simulink model "bpsk_rx_phase_sync"  (R2019a)
settings: Solver=VariableStepAuto  StartTime=0.0  StopTime=4000/3.2e6  RelTol=1e-3
InitFcn:
  | setup_bpsk_receiver
undefined symbols (not defined in the file): AXI4, designMultirateFIR, Lite, tx_data, xlfda_numerator
libraries: xbsIndex_r4 x172, dspmlti4 x11, hdlsllib x11, dspswit3 x4, dspsigops x2, commrandsrc3 x1, simulink x1
(part 2 of 3)

== system bpsk_rx_phase_sync/Time Synchronisation/NCC ==
  note: For the Numerically Controlled Clock (NCC), we need to consider
      | the symbol oversample factor and the fractional wordlength
      | of the accumulator.
      |
      | The number of samples per symbol determine the maximum value
      | of the accumulator {ceil(log2(n))+1}.
      |
      | The fractional bits determine the quantisation step (precision),
      | of our accumulator.
      |
      | We add 1 to the error signal at all times, as this is necessary to
      | ensure the accumulator always adds 1. If the error is equal to
      | zero, then the accumulator will increase normally. If there is an
      | error in phase not equal to zero, the accumulator will change to
      | compensate for the phase difference.
  Error : Inport
  AddSub : xbsIndex_r4/AddSub  mode=Addition  use_carryin=off  use_carryout=off  en=off  latency=0  precision=User Defined  arith_type=Unsigned  n_bits=n+44  bin_pt=44  quantization=Truncate  overflow=Wrap  use_behavioral_HDL=off  hw_selection=Fabric  pipelined=off  dbl_ovrd=off  block_type=addsub
  AddSub1 : xbsIndex_r4/AddSub  mode=Addition  use_carryin=off  use_carryout=off  en=off  latency=0  precision=Full  arith_type="Signed  (2's comp)"  n_bits=45  bin_pt=44  quantization=Truncate  overflow=Flag as error  use_behavioral_HDL=off  hw_selection=Fabric  pipelined=off  dbl_ovrd=off  block_type=addsub
  Constant : xbsIndex_r4/Constant  const=1  gui_display_data_type=Fixed-point  arith_type=Unsigned  n_bits=1  bin_pt=0  preci_type=Single  exp_width=8  frac_width=24  explicit_period=off  period=1  equ=P=C  opselect=C  inp2=PCIN>>17  opr=+  inp1=P  carry=CIN  dbl_ovrd=off  block_type=constant
  Register : xbsIndex_r4/Register  init=0  rst=off  en=off  dbl_ovrd=off  block_type=register
  Relational : xbsIndex_r4/Relational  mode=a<b  op_type=Bool  en=off  latency=0  dbl_ovrd=off  block_type=relational
  Strobe : Outport
  wires:
  Register/1 -> AddSub/1, Relational/2
  Relational/1 -> Strobe/1
  AddSub/1 -> Register/1, Relational/1
  AddSub1/1 -> AddSub/2
  Constant/1 -> AddSub1/1
  Error/1 -> AddSub1/2

== system bpsk_rx_phase_sync/Time Synchronisation/Timing Error Detector ==
  Real In : Inport
  Imag In : Inport  Port=2
  AddSub : xbsIndex_r4/AddSub  mode=Subtraction  use_carryin=off  use_carryout=off  en=off  latency=0  precision=Full  arith_type=Unsigned  n_bits=16  bin_pt=14  quantization=Truncate  overflow=Wrap  use_behavioral_HDL=off  hw_selection=Fabric  pipelined=off  dbl_ovrd=off  block_type=addsub
  AddSub1 : xbsIndex_r4/AddSub  mode=Subtraction  use_carryin=off  use_carryout=off  en=off  latency=0  precision=Full  arith_type=Unsigned  n_bits=16  bin_pt=14  quantization=Truncate  overflow=Wrap  use_behavioral_HDL=off  hw_selection=Fabric  pipelined=off  dbl_ovrd=off  block_type=addsub
  AddSub2 : xbsIndex_r4/AddSub  mode=Addition  use_carryin=off  use_carryout=off  en=off  latency=0  precision=Full  arith_type="Signed  (2's comp)"  n_bits=33  bin_pt=25  quantization="Round  (unbiased: +/- Inf)"  overflow=Saturate  use_behavioral_HDL=off  hw_selection=Fabric  pipelined=off  dbl_ovrd=off  block_type=addsub
  Delay : xbsIndex_r4/Delay  rst=off  infoeditControl=Selection of Reset will increase slice count due to use of real FFs and instead of SRLs  en=off  latency=32  reg_retiming=off  dbl_ovrd=off  block_type=delay
  Delay1 : xbsIndex_r4/Delay  rst=off  infoeditControl=Selection of Reset will increase slice count due to use of real FFs and instead of SRLs  en=off  latency=32  reg_retiming=off  dbl_ovrd=off  block_type=delay
  Mult1 : xbsIndex_r4/Mult  precision=Full  arith_type=Unsigned  n_bits=31  bin_pt=28  quantization=Truncate  overflow=Saturate  en=off  latency=0  use_behavioral_HDL=off  opt=Speed  use_embedded=on  optimum_pipeline=off  pipeline=on  dbl_ovrd=off  use_rpm=on  placement_style=Triangular  block_type=mult
  Mult2 : xbsIndex_r4/Mult  precision=Full  arith_type=Unsigned  n_bits=31  bin_pt=28  quantization=Truncate  overflow=Saturate  en=off  latency=0  use_behavioral_HDL=off  opt=Speed  use_embedded=on  optimum_pipeline=off  pipeline=on  dbl_ovrd=off  use_rpm=on  placement_style=Triangular  block_type=mult
  Error : Outport
  wires:
  Real In/1 -> Mult1/1, Mult1/2
  Imag In/1 -> Mult2/1, Mult2/2
  AddSub/1 -> AddSub2/1
  AddSub2/1 -> Error/1
  Delay1/1 -> AddSub1/2
  Mult2/1 -> Delay1/1, AddSub1/1
  AddSub1/1 -> AddSub2/2
  Mult1/1 -> AddSub/1, Delay/1
  Delay/1 -> AddSub/2

== system bpsk_rx_phase_sync/BPSK System/BPSK RX Generation/RRC Receive Filter ==
  Data In : Inport
  Data Type Conversion2 : DataTypeConversion  OutDataTypeStr=fixdt(1,16,14)
  FDATool : xbsIndex_r4/FDATool  block_type=fdatool
      settings: infoedit=FDATool
  FIR Decimation : dspmlti4/FIR Decimation  FilterSource=Dialog parameters  h=xlfda_numerator('FDATool')/(max(xlfda_numerator('FDATool'))*4)  D=4  filtStruct=Direct form  FilterObject=FDECIM  framing=Allow multirate processing  inputOffset=0  outputBufInitCond=0  roundingMode=Floor  overflowMode=off  firstCoeffMode=Binary point scaling  firstCoeffWordLength=16  firstCoeffFracLength=14  firstCoeffDataTypeStr=fixdt(1,16,14)  firstCoeffMin=[]  firstCoeffMax=[]  firstCoeffLastDataTypeStr=fixdt(1,16,14)  outputDataTypeStr=Inherit: Same as accumulator  outputMin=[]  outputMax=[]  outputLastDataTypeStr=Inherit: Same as accumulator
  Data Out : Outport
  wires:
  FIR Decimation/1 -> Data Type Conversion2/1
  Data In/1 -> FIR Decimation/1
  Data Type Conversion2/1 -> Data Out/1

== system bpsk_rx_phase_sync/BPSK System/BPSK TX Generation/DBPSK Modulator ==
  Input : Inport
  Cast To Boolean : DataTypeConversion  OutDataTypeStr=boolean
  Constant : Constant  Value=fi(1, 1, 16, 14)  OutDataTypeStr=fixdt(1,16,14)  SampleTime=-1
  Constant1 : Constant  Value=fi(-1, 1, 16, 14)  OutDataTypeStr=fixdt(1,16,14)  SampleTime=-1
  Constant2 : Constant  Value=0  OutDataTypeStr=Inherit: Inherit via back propagation  SampleTime=-1
  Delay : Delay  DelayLength=1
  Multiport Switch : MultiPortSwitch  DataPortOrder=Zero-based contiguous  Inputs=2  zeroidx=on
  Real-Imag to Complex : RealImagToComplex
  XOR : Logic  Operator=XOR  IconShape=distinctive  AllPortsSameDT=off  OutDataTypeStr=boolean
  Output : Outport
  wires:
  Constant2/1 -> Real-Imag to Complex/2
  Real-Imag to Complex/1 -> Output/1
  Multiport Switch/1 -> Real-Imag to Complex/1
  Constant1/1 -> Multiport Switch/3
  Constant/1 -> Multiport Switch/2
  Input/1 -> Cast To Boolean/1
  Delay/1 -> XOR/1
  XOR/1 -> Multiport Switch/1, Delay/1
  Cast To Boolean/1 -> XOR/2

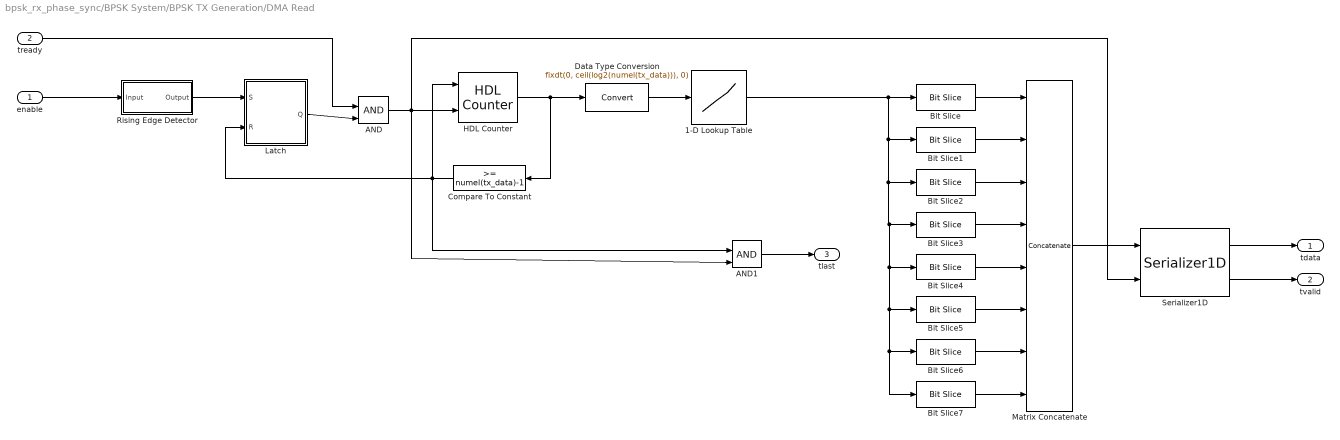
== system bpsk_rx_phase_sync/BPSK System/BPSK TX Generation/DMA Read ==
  enable : Inport
  tready : Inport  Port=2
  1-D Lookup Table : Lookup_n-D  NumberOfTableDimensions=1  BreakpointsForDimension1=[0:1:numel(tx_data)-1]  Table=tx_data  TableDataTypeStr=Inherit: Inherit from 'Table data'  ExtrapMethod=Clip  InternalRulePriority=Speed  OutDataTypeStr=Inherit: Inherit from 'Table data'  RndMeth=Simplest  InputSameDT=on
  AND : Logic  IconShape=distinctive  AllPortsSameDT=off  OutDataTypeStr=boolean
  AND1 : Logic  IconShape=distinctive  AllPortsSameDT=off  OutDataTypeStr=boolean
  Bit Slice : hdlsllib/Logic and Bit Operations/Bit Slice  lidx=0  ridx=0
      settings: SourceProductName=Simulink  SourceProductBaseCode=SL
  Bit Slice1 : hdlsllib/Logic and Bit Operations/Bit Slice  lidx=1  ridx=1
      settings: SourceProductName=Simulink  SourceProductBaseCode=SL
  Bit Slice2 : hdlsllib/Logic and Bit Operations/Bit Slice  lidx=2  ridx=2
      settings: SourceProductName=Simulink  SourceProductBaseCode=SL
  Bit Slice3 : hdlsllib/Logic and Bit Operations/Bit Slice  lidx=3  ridx=3
      settings: SourceProductName=Simulink  SourceProductBaseCode=SL
  Bit Slice4 : hdlsllib/Logic and Bit Operations/Bit Slice  lidx=4  ridx=4
      settings: SourceProductName=Simulink  SourceProductBaseCode=SL
  Bit Slice5 : hdlsllib/Logic and Bit Operations/Bit Slice  lidx=5  ridx=5
      settings: SourceProductName=Simulink  SourceProductBaseCode=SL
  Bit Slice6 : hdlsllib/Logic and Bit Operations/Bit Slice  lidx=6  ridx=6
      settings: SourceProductName=Simulink  SourceProductBaseCode=SL
  Bit Slice7 : hdlsllib/Logic and Bit Operations/Bit Slice  lidx=7  ridx=7
      settings: SourceProductName=Simulink  SourceProductBaseCode=SL
  Compare To Constant : simulink/Logic and Bit Operations/Compare To Constant  relop=>=  const=numel(tx_data)-1  OutDataTypeStr=boolean
  Data Type Conversion : DataTypeConversion  OutDataTypeStr=fixdt(0, ceil(log2(numel(tx_data))), 0)
  HDL Counter : hdlsllib/Sources/HDL Counter  CountType=Free running  CountInit=0  CountStep=1  CountMax=25  CountFromType=Initial value  CountFrom=0  CountResetPort=on  CountLoadPort=off  CountEnbPort=on  CountDirPort=off  CountDataType=Unsigned  CountWordLen=32  CountFracLen=0  CountSampTime=1
      settings: SourceProductName=Simulink
  Latch : Subsystem
  Matrix Concatenate : Concatenate  NumInputs=8  Mode=Multidimensional array  ConcatenateDimension=2
  Rising Edge Detector : Subsystem
  Serializer1D : hdlsllib/HDL Operations/Serializer1D  Ratio=8  IdleCycles=0  validIn=on  startOut=off  validOut=on  inputDataDimensions=-1  inputSampleTime=-1  inputSignalType=auto
      settings: SourceProductName=Simulink  SourceProductBaseCode=SL
  tdata : Outport
  tvalid : Outport  Port=2
  tlast : Outport  Port=3
  wires:
  Serializer1D/2 -> tvalid/1
  Bit Slice5/1 -> Matrix Concatenate/6
  Bit Slice6/1 -> Matrix Concatenate/7
  Bit Slice7/1 -> Matrix Concatenate/8
  Bit Slice4/1 -> Matrix Concatenate/5
  Serializer1D/1 -> tdata/1
  1-D Lookup Table/1 -> Bit Slice/1, Bit Slice1/1, Bit Slice2/1, Bit Slice3/1, Bit Slice4/1, Bit Slice5/1, Bit Slice6/1, Bit Slice7/1
  Bit Slice2/1 -> Matrix Concatenate/3
  Bit Slice1/1 -> Matrix Concatenate/2
  Bit Slice3/1 -> Matrix Concatenate/4
  Bit Slice/1 -> Matrix Concatenate/1
  Matrix Concatenate/1 -> Serializer1D/1
  Compare To Constant/1 -> AND1/1, HDL Counter/1, Latch/2(R)
  enable/1 -> Rising Edge Detector/1(Input)
  HDL Counter/1 -> Compare To Constant/1, Data Type Conversion/1
  Data Type Conversion/1 -> 1-D Lookup Table/1
  Rising Edge Detector/1(Output) -> Latch/1(S)
  AND/1 -> AND1/2, Serializer1D/2, HDL Counter/2
  Latch/1(Q) -> AND/2
  tready/1 -> AND/1
  AND1/1 -> tlast/1

== system bpsk_rx_phase_sync/BPSK System/RF-ADC/Decimation Filter ==
  Data In : Inport
  FIR 0 : dspmlti4/FIR Decimation  FilterSource=Filter object  h=designMultirateFIR(1,2)  D=2  filtStruct=Direct form  FilterObject=fir0  InputProcessing=Columns as channels (frame based)  framing=Allow multirate processing  inputOffset=0  outputBufInitCond=0  roundingMode=Floor  overflowMode=off  firstCoeffDataTypeStr=Inherit: Same word length as input  firstCoeffMin=[]  firstCoeffMax=[]  firstCoeffLastDataTypeStr=Inherit: Same word length as input  outputDataTypeStr=Inherit: Same as accumulator  outputMin=[]  outputMax=[]  outputLastDataTypeStr=Inherit: Same as accumulator
  FIR 1 : dspmlti4/FIR Decimation  FilterSource=Filter object  h=designMultirateFIR(1,2)  D=2  filtStruct=Direct form  FilterObject=fir1  InputProcessing=Columns as channels (frame based)  framing=Allow multirate processing  inputOffset=0  outputBufInitCond=0  roundingMode=Floor  overflowMode=off  firstCoeffDataTypeStr=Inherit: Same word length as input  firstCoeffMin=[]  firstCoeffMax=[]  firstCoeffLastDataTypeStr=Inherit: Same word length as input  outputDataTypeStr=Inherit: Same as accumulator  outputMin=[]  outputMax=[]  outputLastDataTypeStr=Inherit: Same as accumulator
  FIR 2 : dspmlti4/FIR Decimation  FilterSource=Filter object  h=designMultirateFIR(1,2)  D=2  filtStruct=Direct form  FilterObject=fir2  InputProcessing=Columns as channels (frame based)  framing=Allow multirate processing  inputOffset=0  outputBufInitCond=0  roundingMode=Floor  overflowMode=off  firstCoeffDataTypeStr=Inherit: Same word length as input  firstCoeffMin=[]  firstCoeffMax=[]  firstCoeffLastDataTypeStr=Inherit: Same word length as input  outputDataTypeStr=Inherit: Same as accumulator  outputMin=[]  outputMax=[]  outputLastDataTypeStr=Inherit: Same as accumulator
  Data Out : Outport
  wires:
  FIR 2/1 -> FIR 1/1
  Data In/1 -> FIR 2/1
  FIR 0/1 -> Data Out/1
  FIR 1/1 -> FIR 0/1

== system bpsk_rx_phase_sync/BPSK System/RF-ADC/NCO and Mixer ==
  Data In : Inport
  Constant1 : Constant  Value=m  OutDataTypeStr=fixdt(0,2,0)  SampleTime=-1
  Data Type Conversion : DataTypeConversion  OutDataTypeStr=fixdt(1,16,14)
  Multiport Switch1 : MultiPortSwitch  DataPortOrder=Zero-based contiguous  zeroidx=on
  RF-ADC Coarse Mixer : Subsystem
  RF-ADC Fine Mixer : Subsystem
  Real-Imag to Complex : RealImagToComplex
  Data Out : Outport
  wires:
  Data Type Conversion/1 -> Multiport Switch1/2
  Constant1/1 -> Multiport Switch1/1
  Data In/1 -> Real-Imag to Complex/2, RF-ADC Fine Mixer/1(Data In), RF-ADC Coarse Mixer/1(Data In), Real-Imag to Complex/1
  RF-ADC Coarse Mixer/1(Data Out) -> Multiport Switch1/3
  Real-Imag to Complex/1 -> Data Type Conversion/1
  RF-ADC Fine Mixer/1(Data Out) -> Multiport Switch1/4
  Multiport Switch1/1 -> Data Out/1

== system bpsk_rx_phase_sync/BPSK System/RF-ADC/RF-ADC ==
  Data In : Inport
  Buffer : Buffer  N=ssr  OutputFrames=off
  Data Type Conversion : DataTypeConversion  OutDataTypeStr=fixdt(1,12,10)
  Rate Transition : RateTransition  OutPortSampleTime=1/fs
  Data Out : Outport
  wires:
  Buffer/1 -> Data Out/1
  Data Type Conversion/1 -> Buffer/1
  Data In/1 -> Rate Transition/1
  Rate Transition/1 -> Data Type Conversion/1

== system bpsk_rx_phase_sync/BPSK System/RF-DAC/Coarse Delay ==
  Data In : Inport
  Data Out : Outport
  wires:
  Data In/1 -> Data Out/1

== system bpsk_rx_phase_sync/BPSK System/RF-DAC/Interpolation Filter ==
  Data In : Inport
  FIR 0 : dspmlti4/FIR Interpolation  FilterSource=Filter object  h=designMultirateFIR(3,1)  L=2  FilterObject=fir0  InputProcessing=Columns as channels (frame based)  framing=Allow multirate processing  outputBufInitCond=0  roundingMode=Floor  overflowMode=off  firstCoeffDataTypeStr=Inherit: Same word length as input  firstCoeffMin=[]  firstCoeffMax=[]  firstCoeffLastDataTypeStr=Inherit: Same word length as input  outputDataTypeStr=Inherit: Same as accumulator  outputMin=[]  outputMax=[]  outputLastDataTypeStr=Inherit: Same as accumulator
      settings: SourceProductName=DSP System Toolbox
  FIR 1 : dspmlti4/FIR Interpolation  FilterSource=Filter object  h=designMultirateFIR(3,1)  L=2  FilterObject=fir1  InputProcessing=Columns as channels (frame based)  framing=Allow multirate processing  outputBufInitCond=0  roundingMode=Floor  overflowMode=off  firstCoeffDataTypeStr=Inherit: Same word length as input  firstCoeffMin=[]  firstCoeffMax=[]  firstCoeffLastDataTypeStr=Inherit: Same word length as input  outputDataTypeStr=Inherit: Same as accumulator  outputMin=[]  outputMax=[]  outputLastDataTypeStr=Inherit: Same as accumulator
      settings: SourceProductName=DSP System Toolbox
  FIR 2 : dspmlti4/FIR Interpolation  FilterSource=Filter object  h=designMultirateFIR(3,1)  L=2  FilterObject=fir2  InputProcessing=Columns as channels (frame based)  framing=Allow multirate processing  outputBufInitCond=0  roundingMode=Floor  overflowMode=off  firstCoeffDataTypeStr=Inherit: Same word length as input  firstCoeffMin=[]  firstCoeffMax=[]  firstCoeffLastDataTypeStr=Inherit: Same word length as input  outputDataTypeStr=Inherit: Same as accumulator  outputMin=[]  outputMax=[]  outputLastDataTypeStr=Inherit: Same as accumulator
      settings: SourceProductName=DSP System Toolbox
  Data Out : Outport
  wires:
  FIR 1/1 -> FIR 0/1
  FIR 0/1 -> Data Out/1
  Data In/1 -> FIR 2/1
  FIR 2/1 -> FIR 1/1

== system bpsk_rx_phase_sync/BPSK System/RF-DAC/NCO and Mixer ==
  Data In : Inport
  Complex to Real-Imag : ComplexToRealImag
  Constant1 : Constant  Value=m  OutDataTypeStr=fixdt(0,2,0)  SampleTime=-1
  Multiport Switch1 : MultiPortSwitch  DataPortOrder=Zero-based contiguous  zeroidx=on
  RF-DAC Coarse Mixer : Subsystem
  RF-DAC Fine Mixer : Subsystem
  Terminator : Terminator
  Data Out : Outport
  wires:
  Complex to Real-Imag/2 -> Terminator/1
  Complex to Real-Imag/1 -> Multiport Switch1/2
  RF-DAC Fine Mixer/1(Data Out) -> Multiport Switch1/4
  Multiport Switch1/1 -> Data Out/1
  Data In/1 -> RF-DAC Fine Mixer/1(Data In), RF-DAC Coarse Mixer/1(Data In), Complex to Real-Imag/1
  Constant1/1 -> Multiport Switch1/1
  RF-DAC Coarse Mixer/1(Data Out) -> Multiport Switch1/3

== system bpsk_rx_phase_sync/BPSK System/RF-DAC/Output Filter ==
  Data In : Inport
  Data Out : Outport
  wires:
  Data In/1 -> Data Out/1

== system bpsk_rx_phase_sync/BPSK System/RF-DAC/QMC Gain & Phase ==
  Data In : Inport
  Data Out : Outport
  wires:
  Data In/1 -> Data Out/1

== system bpsk_rx_phase_sync/BPSK System/RF-DAC/QMC Threshold ==
  Data In : Inport
  Data Out : Outport
  wires:
  Data In/1 -> Data Out/1

== system bpsk_rx_phase_sync/BPSK System/RF-DAC/RF-DAC ==
  Data In : Inport
  Cast To Double : DataTypeConversion  OutDataTypeStr=double
  Rate Transition : RateTransition  OutPortSampleTime=0
  Unbuffer : Unbuffer
  Data Out : Outport
  wires:
  Rate Transition/1 -> Data Out/1
  Data In/1 -> Unbuffer/1
  Unbuffer/1 -> Cast To Double/1
  Cast To Double/1 -> Rate Transition/1

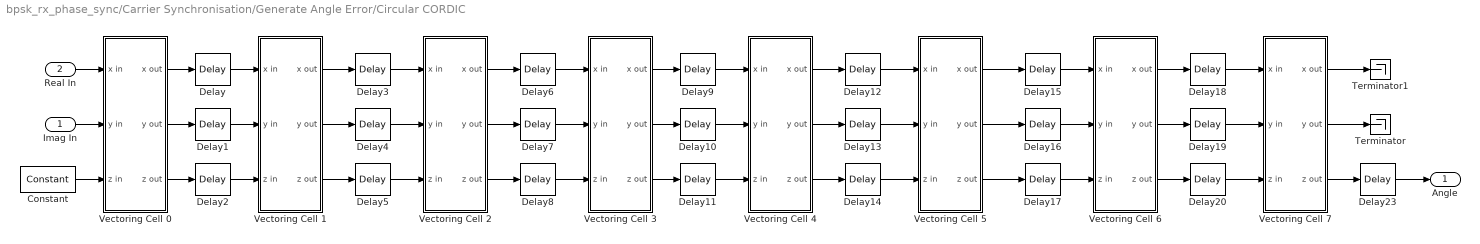
== system bpsk_rx_phase_sync/Carrier Synchronisation/Generate Angle Error/Circular CORDIC ==
  Imag In : Inport
  Real In : Inport  Port=2
  Constant : xbsIndex_r4/Constant  const=0  gui_display_data_type=Fixed-point  arith_type=Signed (2's comp)  n_bits=16  bin_pt=14  preci_type=Single  exp_width=8  frac_width=24  explicit_period=off  period=1  equ=P=C  opselect=C  inp2=PCIN>>17  opr=+  inp1=P  carry=CIN  dbl_ovrd=off  block_type=constant
  Delay{,1..20,23} (22 alike) : xbsIndex_r4/Delay  rst=off  infoeditControl=Selection of Reset will increase slice count due to use of real FFs and instead of SRLs  en=off  latency=1  reg_retiming=off  dbl_ovrd=off  block_type=delay
  Terminator : Terminator
  Terminator1 : Terminator
  Vectoring Cell 0 : Subsystem  mask(Cordic Vectoring Cell){i=0}
      mask prompts: i "Iteration:"
      mask help: some notes to go here
      mask DialogControl DescGroupVar Prompt: CORDIC Vectoring Cell
      mask DialogControl DescTextVar Prompt: A single cell of a vectoring CORDIC unrolled architecture.
      mask DialogControl ParameterGroupVar Prompt: Main
  Vectoring Cell 1 : Subsystem  mask(Cordic Vectoring Cell){i=1}
      mask prompts: i "Iteration:"
      mask help: some notes to go here
      mask DialogControl DescGroupVar Prompt: CORDIC Vectoring Cell
      mask DialogControl DescTextVar Prompt: A single cell of a vectoring CORDIC unrolled architecture.
      mask DialogControl ParameterGroupVar Prompt: Main
  Vectoring Cell 2 : Subsystem  mask(Cordic Vectoring Cell){i=2}
      mask prompts: i "Iteration:"
      mask help: some notes to go here
      mask DialogControl DescGroupVar Prompt: CORDIC Vectoring Cell
      mask DialogControl DescTextVar Prompt: A single cell of a vectoring CORDIC unrolled architecture.
      mask DialogControl ParameterGroupVar Prompt: Main
  Vectoring Cell 3 : Subsystem  mask(Cordic Vectoring Cell){i=3}
      mask prompts: i "Iteration:"
      mask help: some notes to go here
      mask DialogControl DescGroupVar Prompt: CORDIC Vectoring Cell
      mask DialogControl DescTextVar Prompt: A single cell of a vectoring CORDIC unrolled architecture.
      mask DialogControl ParameterGroupVar Prompt: Main
  Vectoring Cell 4 : Subsystem  mask(Cordic Vectoring Cell){i=4}
      mask prompts: i "Iteration:"
      mask help: some notes to go here
      mask DialogControl DescGroupVar Prompt: CORDIC Vectoring Cell
      mask DialogControl DescTextVar Prompt: A single cell of a vectoring CORDIC unrolled architecture.
      mask DialogControl ParameterGroupVar Prompt: Main
  Vectoring Cell 5 : Subsystem  mask(Cordic Vectoring Cell){i=5}
      mask prompts: i "Iteration:"
      mask help: some notes to go here
      mask DialogControl DescGroupVar Prompt: CORDIC Vectoring Cell
      mask DialogControl DescTextVar Prompt: A single cell of a vectoring CORDIC unrolled architecture.
      mask DialogControl ParameterGroupVar Prompt: Main
  Vectoring Cell 6 : Subsystem  mask(Cordic Vectoring Cell){i=6}
      mask prompts: i "Iteration:"
      mask help: some notes to go here
      mask DialogControl DescGroupVar Prompt: CORDIC Vectoring Cell
      mask DialogControl DescTextVar Prompt: A single cell of a vectoring CORDIC unrolled architecture.
      mask DialogControl ParameterGroupVar Prompt: Main
  Vectoring Cell 7 : Subsystem  mask(Cordic Vectoring Cell){i=7}
      mask prompts: i "Iteration:"
      mask help: some notes to go here
      mask DialogControl DescGroupVar Prompt: CORDIC Vectoring Cell
      mask DialogControl DescTextVar Prompt: A single cell of a vectoring CORDIC unrolled architecture.
      mask DialogControl ParameterGroupVar Prompt: Main
  Angle : Outport
  wires:
  Vectoring Cell 6/3(z out) -> Delay20/1
  Delay5/1 -> Vectoring Cell 2/3(z in)
  Vectoring Cell 6/2(y out) -> Delay19/1
  Vectoring Cell 2/1(x out) -> Delay6/1
  Vectoring Cell 1/3(z out) -> Delay5/1
  Delay14/1 -> Vectoring Cell 5/3(z in)
  Delay20/1 -> Vectoring Cell 7/3(z in)
  Delay15/1 -> Vectoring Cell 6/1(x in)
  Delay7/1 -> Vectoring Cell 3/2(y in)
  Delay1/1 -> Vectoring Cell 1/2(y in)
  Vectoring Cell 3/1(x out) -> Delay9/1
  Delay13/1 -> Vectoring Cell 5/2(y in)
  Delay9/1 -> Vectoring Cell 4/1(x in)
  Vectoring Cell 1/1(x out) -> Delay3/1
  Delay16/1 -> Vectoring Cell 6/2(y in)
  Delay18/1 -> Vectoring Cell 7/1(x in)
  Vectoring Cell 0/3(z out) -> Delay2/1
  Delay10/1 -> Vectoring Cell 4/2(y in)
  Vectoring Cell 2/2(y out) -> Delay7/1
  Vectoring Cell 3/3(z out) -> Delay11/1
  Delay6/1 -> Vectoring Cell 3/1(x in)
  Delay19/1 -> Vectoring Cell 7/2(y in)
  Delay4/1 -> Vectoring Cell 2/2(y in)
  Delay3/1 -> Vectoring Cell 2/1(x in)
  Vectoring Cell 4/3(z out) -> Delay14/1
  Delay8/1 -> Vectoring Cell 3/3(z in)
  Vectoring Cell 3/2(y out) -> Delay10/1
  Vectoring Cell 1/2(y out) -> Delay4/1
  Vectoring Cell 5/1(x out) -> Delay15/1
  Delay/1 -> Vectoring Cell 1/1(x in)
  Vectoring Cell 5/2(y out) -> Delay16/1
  Vectoring Cell 0/1(x out) -> Delay/1
  Vectoring Cell 2/3(z out) -> Delay8/1
  Vectoring Cell 6/1(x out) -> Delay18/1
  Vectoring Cell 0/2(y out) -> Delay1/1
  Delay12/1 -> Vectoring Cell 5/1(x in)
  Vectoring Cell 4/2(y out) -> Delay13/1
  Vectoring Cell 4/1(x out) -> Delay12/1
  Delay2/1 -> Vectoring Cell 1/3(z in)
  Vectoring Cell 5/3(z out) -> Delay17/1
  Delay17/1 -> Vectoring Cell 6/3(z in)
  Delay11/1 -> Vectoring Cell 4/3(z in)
  Vectoring Cell 7/3(z out) -> Delay23/1
  Real In/1 -> Vectoring Cell 0/1(x in)
  Imag In/1 -> Vectoring Cell 0/2(y in)
  Constant/1 -> Vectoring Cell 0/3(z in)
  Delay23/1 -> Angle/1
  Vectoring Cell 7/2(y out) -> Terminator/1
  Vectoring Cell 7/1(x out) -> Terminator1/1

== system bpsk_rx_phase_sync/Carrier Synchronisation/Generate NCO/Loop Filter ==
  Signal : Inport
  Strobe : Inport  Port=2
  Reset : Inport  Port=3
  AddSub : xbsIndex_r4/AddSub  mode=Addition  use_carryin=off  use_carryout=off  en=off  latency=0  precision=User Defined  arith_type="Signed  (2's comp)"  n_bits=36  bin_pt=34  quantization=Truncate  overflow=Flag as error  use_behavioral_HDL=off  hw_selection=Fabric  pipelined=off  dbl_ovrd=off  block_type=addsub
  AddSub1 : xbsIndex_r4/AddSub  mode=Addition  use_carryin=off  use_carryout=off  en=off  latency=0  precision=Full  arith_type="Signed  (2's comp)"  n_bits=32  bin_pt=31  quantization=Truncate  overflow=Wrap  use_behavioral_HDL=off  hw_selection=Fabric  pipelined=off  dbl_ovrd=off  block_type=addsub
  K1_Gain : xbsIndex_r4/CMult  const=K1  gui_display_data_type=Fixed-point  const_n_bits=16  const_bin_pt=16  float_type=Single  exp_bits=8  fraction_bits=24  en=off  latency=0  precision=Full  arith_type="Signed  (2's comp)"  n_bits=20  bin_pt=14  quantization=Truncate  overflow=Wrap  use_behavioral_HDL=off  mem_type=Distributed RAM  pipeline=off  dbl_ovrd=off  block_type=cmult
  K2_Gain : xbsIndex_r4/CMult  const=K2  gui_display_data_type=Fixed-point  const_n_bits=16  const_bin_pt=16  float_type=Single  exp_bits=8  fraction_bits=24  en=off  latency=0  precision=Full  arith_type="Signed  (2's comp)"  n_bits=20  bin_pt=14  quantization=Truncate  overflow=Wrap  use_behavioral_HDL=off  mem_type=Distributed RAM  pipeline=off  dbl_ovrd=off  block_type=cmult
  Register : xbsIndex_r4/Register  init=0  rst=on  en=on  dbl_ovrd=off  block_type=register
  Register1 : xbsIndex_r4/Register  init=0  rst=on  en=on  dbl_ovrd=off  block_type=register
  Register3 : xbsIndex_r4/Register  init=0  rst=off  en=off  dbl_ovrd=off  block_type=register
  Register4 : xbsIndex_r4/Register  init=0  rst=off  en=off  dbl_ovrd=off  block_type=register
  Error : Outport
  Valid : Outport  Port=2
  wires:
  Reset/1 -> Register/2, Register1/2
  Signal/1 -> Register1/1
  K2_Gain/1 -> AddSub/1
  AddSub/1 -> AddSub1/2, Register/1
  Register/1 -> AddSub/2
  Register1/1 -> K2_Gain/1, K1_Gain/1
  AddSub1/1 -> Register3/1
  K1_Gain/1 -> AddSub1/1
  Register3/1 -> Error/1
  Register4/1 -> Valid/1
  Strobe/1 -> Register4/1, Register/3, Register1/3

== system bpsk_rx_phase_sync/Carrier Synchronisation/Generate NCO/NCO ==
  Step Size : Inport
  En_in : Inport  Port=2
  AddSub4 : xbsIndex_r4/AddSub  mode=Addition  use_carryin=off  use_carryout=off  en=off  latency=0  precision=User Defined  arith_type="Signed  (2's comp)"  n_bits=n+b  bin_pt=b  quantization=Truncate  overflow=Wrap  use_behavioral_HDL=off  hw_selection=Fabric  pipelined=off  dbl_ovrd=off  block_type=addsub
  CMult1 : xbsIndex_r4/CMult  const=(2^n)/(2*pi)  gui_display_data_type=Fixed-point  const_n_bits=k_n+b  const_bin_pt=b  float_type=Single  exp_bits=8  fraction_bits=24  en=off  latency=0  precision=User Defined  arith_type="Signed  (2's comp)"  n_bits=n+b  bin_pt=b  quantization=Truncate  overflow=Wrap  use_behavioral_HDL=off  mem_type=Distributed RAM  pipeline=off  dbl_ovrd=off  block_type=cmult
  Convert1 : xbsIndex_r4/Convert  gui_display_data_type=Fixed-point  arith_type=Unsigned  n_bits=n  bin_pt=0  float_type=Single  exp_bits=8  fraction_bits=24  quantization=Truncate  overflow=Wrap  en=off  latency=0  pipeline=off  dbl_ovrd=off  block_type=convert
  Cos ROM : xbsIndex_r4/ROM  depth=2^n  initVector=cos(pi*(0:((2^n)-1))/(2^(n-1)))  distributed_mem=Block RAM  rst=off  init_reg=0  en=off  latency=1  gui_display_data_type=Fixed-point  arith_type="Signed  (2's comp)"  n_bits=16  bin_pt=14  preci_type=Single  exp_width=8  frac_width=24  optimize=Area  use_rpm=on  dbl_ovrd=off  block_type=sprom
  Neg Sin ROM : xbsIndex_r4/ROM  depth=2^n  initVector=-sin(pi*(0:((2^n)-1))/(2^(n-1)))  distributed_mem=Block RAM  rst=off  init_reg=0  en=off  latency=1  gui_display_data_type=Fixed-point  arith_type="Signed  (2's comp)"  n_bits=16  bin_pt=14  preci_type=Single  exp_width=8  frac_width=24  optimize=Area  use_rpm=on  dbl_ovrd=off  block_type=sprom
  Register : xbsIndex_r4/Register  init=0  rst=off  en=off  dbl_ovrd=off  block_type=register
  Register1 : xbsIndex_r4/Register  init=0  rst=off  en=on  dbl_ovrd=off  block_type=register
  Cos : Outport
  Neg Sin : Outport  Port=2
  En_out : Outport  Port=3
  wires:
  Convert1/1 -> Neg Sin ROM/1, Cos ROM/1
  AddSub4/1 -> Register1/1, Convert1/1
  Neg Sin ROM/1 -> Neg Sin/1
  Register1/1 -> AddSub4/2
  CMult1/1 -> AddSub4/1
  Step Size/1 -> CMult1/1
  En_in/1 -> Register/1, Register1/2
  Cos ROM/1 -> Cos/1
  Register/1 -> En_out/1

== system bpsk_rx_phase_sync/BPSK System/BPSK TX Generation/DMA Read/Latch ==
  S : Inport
  R : Inport  Port=2
  Multiport Switch : MultiPortSwitch  DataPortOrder=Zero-based contiguous  Inputs=2  zeroidx=on
  Unit Delay Resettable Synchronous : hdlsllib/Discrete/Unit Delay Resettable Synchronous  InitialCondition=0.0  SampleTime=-1
      settings: SourceProductName=Simulink  SourceProductBaseCode=SL
  Q : Outport
  wires:
  Multiport Switch/1 -> Unit Delay Resettable Synchronous/1, Q/1
  S/1 -> Multiport Switch/3, Multiport Switch/1
  Unit Delay Resettable Synchronous/1 -> Multiport Switch/2
  R/1 -> Unit Delay Resettable Synchronous/2

== system bpsk_rx_phase_sync/BPSK System/BPSK TX Generation/DMA Read/Rising Edge Detector ==
  Input : Inport
  AND1 : Logic  IconShape=distinctive  AllPortsSameDT=off  OutDataTypeStr=boolean
  Delay1 : Delay  DelayLength=1
  NOT : Logic  Operator=NOT  IconShape=distinctive  AllPortsSameDT=off  OutDataTypeStr=boolean
  Output : Outport
  wires:
  NOT/1 -> AND1/1
  Input/1 -> AND1/2, Delay1/1
  Delay1/1 -> NOT/1
  AND1/1 -> Output/1

== system bpsk_rx_phase_sync/BPSK System/RF-ADC/NCO and Mixer/RF-ADC Coarse Mixer ==
  Data In : Inport
  Constant : Constant  Value=mc  OutDataTypeStr=fixdt(0,2,0)  SampleTime=-1
  Data Type Conversion : DataTypeConversion  OutDataTypeStr=fixdt(1,16,14)
  Multiport Switch1 : MultiPortSwitch  DataPortOrder=Zero-based contiguous  zeroidx=on
  Negate : Subsystem
  fs_2 : Subsystem
  fs_4 : Subsystem
  Data Out : Outport
  wires:
  Data Type Conversion/1 -> Data Out/1
  fs_4/1(Data Out) -> Multiport Switch1/3, Negate/1(Data In)
  Negate/1(Data Out) -> Multiport Switch1/4
  Data In/1 -> fs_2/1(Data In), fs_4/1(Data In)
  Constant/1 -> Multiport Switch1/1
  fs_2/1(Data Out) -> Multiport Switch1/2
  Multiport Switch1/1 -> Data Type Conversion/1

== system bpsk_rx_phase_sync/BPSK System/RF-ADC/NCO and Mixer/RF-ADC Fine Mixer ==
  Data In : Inport
  Complex to Real-Imag : ComplexToRealImag
  Constant : Constant  Value=0  SampleTime=-1
  Multiport Switch : MultiPortSwitch  DataPortOrder=Zero-based contiguous  Inputs=2  zeroidx=on
  NCO : dspsigops/NCO  AccIncSrc=Specify via dialog  AccInc=fix((((fc*1e9)*(2^18))/(fs))*2^30)  PhaseOffsetSrc=Specify via dialog  PhaseOffset=fix((((2^18)*fph)/(2*pi))*2^30)  AccumWL=48  HasDither=off  DitherWL=4  PNgeneratorLength=19  HasPhaseQuantizer=on  TableDepth=18  HasOutputPhaseError=off  Formula=Sine and cosine  DataType=Binary point scaling  OutputWL=16  OutputFL=14  CompMethod=Table lookup (no interpolation)  SampleTime=1/(fs)  SamplesPerFrame=ssr  OutputFrames=off
      settings: SourceProductName=DSP System Toolbox  SourceProductBaseCode=DS
  Product : Product  OutDataTypeStr=fixdt(1,16,14)
  Product1 : Product  OutDataTypeStr=fixdt(1,16,14)
  Real-Imag to Complex : RealImagToComplex
  Real-Imag to Complex1 : RealImagToComplex
  Shift Arithmetic : ArithShift  BitShiftNumber=1  BitShiftDirection=Right
  Shift Arithmetic1 : ArithShift  BitShiftNumber=1  BitShiftDirection=Right
  Data Out : Outport
  wires:
  Product/1 -> Real-Imag to Complex/2
  Product1/1 -> Real-Imag to Complex/1
  Real-Imag to Complex/1 -> Complex to Real-Imag/1, Multiport Switch/2
  NCO/2 -> Product1/2
  NCO/1 -> Product/2
  Real-Imag to Complex1/1 -> Multiport Switch/3
  Shift Arithmetic/1 -> Real-Imag to Complex1/2
  Shift Arithmetic1/1 -> Real-Imag to Complex1/1
  Complex to Real-Imag/1 -> Shift Arithmetic1/1
  Complex to Real-Imag/2 -> Shift Arithmetic/1
  Multiport Switch/1 -> Data Out/1
  Constant/1 -> Multiport Switch/1
  Data In/1 -> Product/1, Product1/1

== system bpsk_rx_phase_sync/BPSK System/RF-DAC/NCO and Mixer/RF-DAC Coarse Mixer ==
  Data In : Inport
  Add2 : Sum
  Complex to Real-Imag : ComplexToRealImag
  Constant : Constant  Value=mc  OutDataTypeStr=fixdt(0,2,0)  SampleTime=-1
  Multiport Switch1 : MultiPortSwitch  DataPortOrder=Zero-based contiguous  zeroidx=on
  Negate : Subsystem
  fs_2 : Subsystem
  fs_4 : Subsystem
  Data Out : Outport
  wires:
  Add2/1 -> Data Out/1
  Complex to Real-Imag/2 -> Add2/2
  Complex to Real-Imag/1 -> Add2/1
  Multiport Switch1/1 -> Complex to Real-Imag/1
  fs_2/1(Data Out) -> Multiport Switch1/2
  Constant/1 -> Multiport Switch1/1
  Data In/1 -> fs_4/1(Data In), fs_2/1(Data In)
  Negate/1(Data Out) -> Multiport Switch1/4
  fs_4/1(Data Out) -> Negate/1(Data In), Multiport Switch1/3

== system bpsk_rx_phase_sync/BPSK System/RF-DAC/NCO and Mixer/RF-DAC Fine Mixer ==
  Data In : Inport
  Add2 : Sum
  Complex to Real-Imag1 : ComplexToRealImag
  Constant : Constant  Value=0  OutDataTypeStr=boolean  SampleTime=-1
  Multiport Switch : MultiPortSwitch  DataPortOrder=Zero-based contiguous  Inputs=2  zeroidx=on
  NCO : dspsigops/NCO  AccIncSrc=Specify via dialog  AccInc=fix((((fc*1e9)*(2^18))/(fs))*2^30)  PhaseOffsetSrc=Specify via dialog  PhaseOffset=fix((((2^18)*fph)/(2*pi))*2^30)  AccumWL=48  HasDither=off  DitherWL=4  PNgeneratorLength=19  HasPhaseQuantizer=on  TableDepth=18  HasOutputPhaseError=off  Formula=Sine and cosine  DataType=Binary point scaling  OutputWL=16  OutputFL=14  CompMethod=Table lookup (no interpolation)  SampleTime=1/(fs)  SamplesPerFrame=ssr  OutputFrames=off
      settings: SourceProductName=DSP System Toolbox  SourceProductBaseCode=DS
  Product1 : Product  OutDataTypeStr=Inherit: Same as first input
  Product4 : Product  OutDataTypeStr=Inherit: Same as first input
  Shift Arithmetic1 : ArithShift  BitShiftNumber=1  BitShiftDirection=Right
  Data Out : Outport
  wires:
  Product1/1 -> Add2/2
  Complex to Real-Imag1/2 -> Product4/1
  Complex to Real-Imag1/1 -> Product1/2
  NCO/2 -> Product1/1
  NCO/1 -> Product4/2
  Product4/1 -> Add2/1
  Data In/1 -> Complex to Real-Imag1/1
  Constant/1 -> Multiport Switch/1
  Multiport Switch/1 -> Data Out/1
  Add2/1 -> Shift Arithmetic1/1, Multiport Switch/2
  Shift Arithmetic1/1 -> Multiport Switch/3

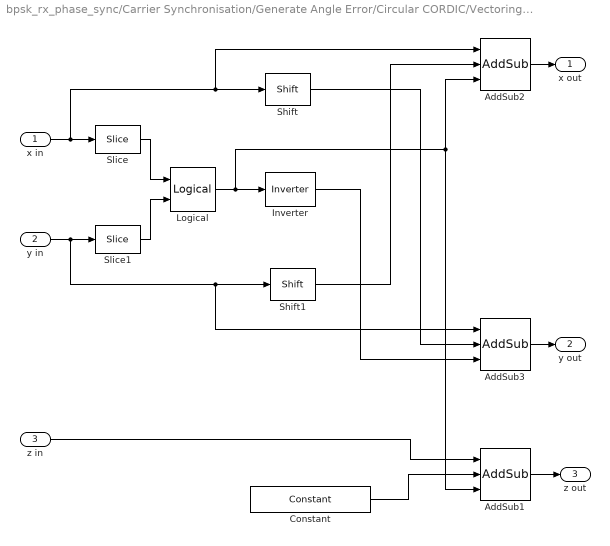
== system bpsk_rx_phase_sync/Carrier Synchronisation/Generate Angle Error/Circular CORDIC/Vectoring Cell 0 ==
  x in : Inport
  y in : Inport  Port=2
  z in : Inport  Port=3
  AddSub1 : xbsIndex_r4/AddSub  mode=Addition or Subtraction  use_carryin=off  use_carryout=off  en=off  latency=0  precision=User Defined  arith_type="Signed  (2's comp)"  n_bits=20  bin_pt=18  quantization=Truncate  overflow=Wrap  use_behavioral_HDL=on  hw_selection=Fabric  pipelined=off  use_rpm=on  dbl_ovrd=off  block_type=addsub
      settings: xl_area=[0, 0, 0, 0, 0, 0, 0]  block_version=VER_STRING_GOES_HERE
  AddSub2 : xbsIndex_r4/AddSub  mode=Addition or Subtraction  use_carryin=off  use_carryout=off  en=off  latency=0  precision=User Defined  arith_type="Signed  (2's comp)"  n_bits=15  bin_pt=12  quantization=Truncate  overflow=Wrap  use_behavioral_HDL=on  hw_selection=Fabric  pipelined=off  use_rpm=on  dbl_ovrd=off  block_type=addsub
      settings: xl_area=[0, 0, 0, 0, 0, 0, 0]  block_version=VER_STRING_GOES_HERE
  AddSub3 : xbsIndex_r4/AddSub  mode=Addition or Subtraction  use_carryin=off  use_carryout=off  en=off  latency=0  precision=User Defined  arith_type="Signed  (2's comp)"  n_bits=15  bin_pt=12  quantization=Truncate  overflow=Wrap  use_behavioral_HDL=on  hw_selection=Fabric  pipelined=off  use_rpm=on  dbl_ovrd=off  block_type=addsub
      settings: xl_area=[0, 0, 0, 0, 0, 0, 0]  block_version=VER_STRING_GOES_HERE
  Constant : xbsIndex_r4/Constant  const=atan(2^-i)  gui_display_data_type=Fixed-point  arith_type=Signed (2's comp)  n_bits=20  bin_pt=18  preci_type=Single  exp_width=8  frac_width=24  explicit_period=off  period=1  equ=P=C  opselect=C  inp2=PCIN>>17  opr=+  inp1=P  carry=CIN  dbl_ovrd=off  block_type=constant
      settings: block_version=10.1.2
  Inverter : xbsIndex_r4/Inverter  en=off  latency=0  dbl_ovrd=off  block_type=inv
      settings: xl_area=[0, 0, 0, 0, 0, 0, 0]  block_version=VER_STRING_GOES_HERE
  Logical : xbsIndex_r4/Logical  logical_function=XOR  inputs=2  en=off  latency=0  precision=Full  arith_type=Unsigned  n_bits=1  bin_pt=0  align_bp=on  dbl_ovrd=off  block_type=logical
      settings: xl_area=[0, 0, 0, 0, 0, 0, 0]  block_version=VER_STRING_GOES_HERE
  Shift : xbsIndex_r4/Shift  shift_dir=Right  shift_bits=i  en=off  latency=0  precision=User Defined  arith_type="Signed  (2's comp)"  n_bits=15  bin_pt=12  quantization=Truncate  overflow=Wrap  dbl_ovrd=off  block_type=shift
      settings: xl_area=[0, 0, 0, 0, 0, 0, 0]  block_version=VER_STRING_GOES_HERE
  Shift1 : xbsIndex_r4/Shift  shift_dir=Right  shift_bits=i  en=off  latency=0  precision=User Defined  arith_type="Signed  (2's comp)"  n_bits=15  bin_pt=12  quantization=Truncate  overflow=Wrap  dbl_ovrd=off  block_type=shift
      settings: xl_area=[0, 0, 0, 0, 0, 0, 0]  block_version=VER_STRING_GOES_HERE
  Slice : xbsIndex_r4/Slice  nbits=1  boolean_output=on  mode=Upper Bit Location + Width  bit1=0  base1=MSB of Input  bit0=0  base0=LSB of Input  dbl_ovrd=off  block_type=slice
      settings: infoedit="Extracts a given range of bits from each input sample and presents it at the output.  The output type is ordinarily unsigned with binary point at zero, but can be Boolean when the slice is one bit wide.<P><P>Hardware notes: In hardware this block costs nothing."  block_version=VER_STRING_GOES_HERE
  Slice1 : xbsIndex_r4/Slice  nbits=1  boolean_output=on  mode=Upper Bit Location + Width  bit1=0  base1=MSB of Input  bit0=0  base0=LSB of Input  dbl_ovrd=off  block_type=slice
      settings: infoedit="Extracts a given range of bits from each input sample and presents it at the output.  The output type is ordinarily unsigned with binary point at zero, but can be Boolean when the slice is one bit wide.<P><P>Hardware notes: In hardware this block costs nothing."  block_version=VER_STRING_GOES_HERE
  x out : Outport
  y out : Outport  Port=2
  z out : Outport  Port=3
  wires:
  x in/1 -> AddSub2/1, Shift/1, Slice/1
  y in/1 -> AddSub3/1, Shift1/1, Slice1/1
  Slice/1 -> Logical/1
  Slice1/1 -> Logical/2
  Logical/1 -> Inverter/1, AddSub2/3, AddSub1/3
  Shift1/1 -> AddSub2/2
  Shift/1 -> AddSub3/2
  Inverter/1 -> AddSub3/3
  AddSub2/1 -> x out/1
  AddSub3/1 -> y out/1
  z in/1 -> AddSub1/1
  Constant/1 -> AddSub1/2
  AddSub1/1 -> z out/1

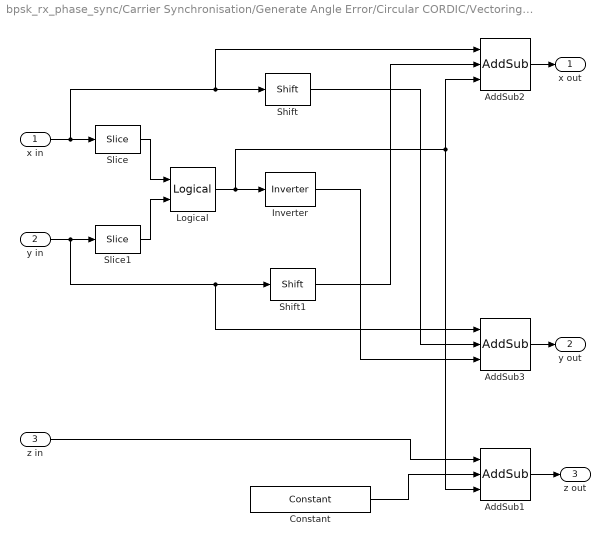
== system bpsk_rx_phase_sync/Carrier Synchronisation/Generate Angle Error/Circular CORDIC/Vectoring Cell 1 ==
  x in : Inport
  y in : Inport  Port=2
  z in : Inport  Port=3
  AddSub1 : xbsIndex_r4/AddSub  mode=Addition or Subtraction  use_carryin=off  use_carryout=off  en=off  latency=0  precision=User Defined  arith_type="Signed  (2's comp)"  n_bits=20  bin_pt=18  quantization=Truncate  overflow=Wrap  use_behavioral_HDL=on  hw_selection=Fabric  pipelined=off  use_rpm=on  dbl_ovrd=off  block_type=addsub
      settings: xl_area=[0, 0, 0, 0, 0, 0, 0]  block_version=VER_STRING_GOES_HERE
  AddSub2 : xbsIndex_r4/AddSub  mode=Addition or Subtraction  use_carryin=off  use_carryout=off  en=off  latency=0  precision=User Defined  arith_type="Signed  (2's comp)"  n_bits=15  bin_pt=12  quantization=Truncate  overflow=Wrap  use_behavioral_HDL=on  hw_selection=Fabric  pipelined=off  use_rpm=on  dbl_ovrd=off  block_type=addsub
      settings: xl_area=[0, 0, 0, 0, 0, 0, 0]  block_version=VER_STRING_GOES_HERE
  AddSub3 : xbsIndex_r4/AddSub  mode=Addition or Subtraction  use_carryin=off  use_carryout=off  en=off  latency=0  precision=User Defined  arith_type="Signed  (2's comp)"  n_bits=15  bin_pt=12  quantization=Truncate  overflow=Wrap  use_behavioral_HDL=on  hw_selection=Fabric  pipelined=off  use_rpm=on  dbl_ovrd=off  block_type=addsub
      settings: xl_area=[0, 0, 0, 0, 0, 0, 0]  block_version=VER_STRING_GOES_HERE
  Constant : xbsIndex_r4/Constant  const=atan(2^-i)  gui_display_data_type=Fixed-point  arith_type=Signed (2's comp)  n_bits=20  bin_pt=18  preci_type=Single  exp_width=8  frac_width=24  explicit_period=off  period=1  equ=P=C  opselect=C  inp2=PCIN>>17  opr=+  inp1=P  carry=CIN  dbl_ovrd=off  block_type=constant
      settings: block_version=10.1.2
  Inverter : xbsIndex_r4/Inverter  en=off  latency=0  dbl_ovrd=off  block_type=inv
      settings: xl_area=[0, 0, 0, 0, 0, 0, 0]  block_version=VER_STRING_GOES_HERE
  Logical : xbsIndex_r4/Logical  logical_function=XOR  inputs=2  en=off  latency=0  precision=Full  arith_type=Unsigned  n_bits=1  bin_pt=0  align_bp=on  dbl_ovrd=off  block_type=logical
      settings: xl_area=[0, 0, 0, 0, 0, 0, 0]  block_version=VER_STRING_GOES_HERE
  Shift : xbsIndex_r4/Shift  shift_dir=Right  shift_bits=i  en=off  latency=0  precision=User Defined  arith_type="Signed  (2's comp)"  n_bits=15  bin_pt=12  quantization=Truncate  overflow=Wrap  dbl_ovrd=off  block_type=shift
      settings: xl_area=[0, 0, 0, 0, 0, 0, 0]  block_version=VER_STRING_GOES_HERE
  Shift1 : xbsIndex_r4/Shift  shift_dir=Right  shift_bits=i  en=off  latency=0  precision=User Defined  arith_type="Signed  (2's comp)"  n_bits=15  bin_pt=12  quantization=Truncate  overflow=Wrap  dbl_ovrd=off  block_type=shift
      settings: xl_area=[0, 0, 0, 0, 0, 0, 0]  block_version=VER_STRING_GOES_HERE
  Slice : xbsIndex_r4/Slice  nbits=1  boolean_output=on  mode=Upper Bit Location + Width  bit1=0  base1=MSB of Input  bit0=0  base0=LSB of Input  dbl_ovrd=off  block_type=slice
      settings: infoedit="Extracts a given range of bits from each input sample and presents it at the output.  The output type is ordinarily unsigned with binary point at zero, but can be Boolean when the slice is one bit wide.<P><P>Hardware notes: In hardware this block costs nothing."  block_version=VER_STRING_GOES_HERE
  Slice1 : xbsIndex_r4/Slice  nbits=1  boolean_output=on  mode=Upper Bit Location + Width  bit1=0  base1=MSB of Input  bit0=0  base0=LSB of Input  dbl_ovrd=off  block_type=slice
      settings: infoedit="Extracts a given range of bits from each input sample and presents it at the output.  The output type is ordinarily unsigned with binary point at zero, but can be Boolean when the slice is one bit wide.<P><P>Hardware notes: In hardware this block costs nothing."  block_version=VER_STRING_GOES_HERE
  x out : Outport
  y out : Outport  Port=2
  z out : Outport  Port=3
  wires:
  AddSub1/1 -> z out/1
  Constant/1 -> AddSub1/2
  z in/1 -> AddSub1/1
  AddSub3/1 -> y out/1
  AddSub2/1 -> x out/1
  Inverter/1 -> AddSub3/3
  Shift/1 -> AddSub3/2
  Shift1/1 -> AddSub2/2
  Logical/1 -> AddSub1/3, AddSub2/3, Inverter/1
  Slice1/1 -> Logical/2
  Slice/1 -> Logical/1
  y in/1 -> Slice1/1, Shift1/1, AddSub3/1
  x in/1 -> Slice/1, Shift/1, AddSub2/1

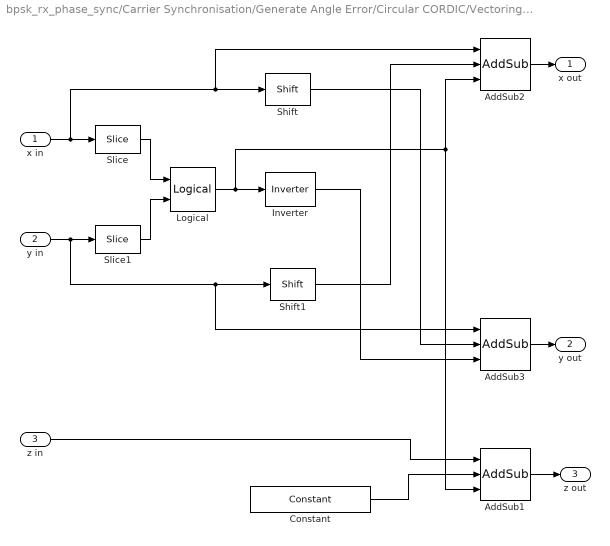
== system bpsk_rx_phase_sync/Carrier Synchronisation/Generate Angle Error/Circular CORDIC/Vectoring Cell 2 ==
  x in : Inport
  y in : Inport  Port=2
  z in : Inport  Port=3
  AddSub1 : xbsIndex_r4/AddSub  mode=Addition or Subtraction  use_carryin=off  use_carryout=off  en=off  latency=0  precision=User Defined  arith_type="Signed  (2's comp)"  n_bits=20  bin_pt=18  quantization=Truncate  overflow=Wrap  use_behavioral_HDL=on  hw_selection=Fabric  pipelined=off  use_rpm=on  dbl_ovrd=off  block_type=addsub
      settings: xl_area=[0, 0, 0, 0, 0, 0, 0]  block_version=VER_STRING_GOES_HERE
  AddSub2 : xbsIndex_r4/AddSub  mode=Addition or Subtraction  use_carryin=off  use_carryout=off  en=off  latency=0  precision=User Defined  arith_type="Signed  (2's comp)"  n_bits=15  bin_pt=12  quantization=Truncate  overflow=Wrap  use_behavioral_HDL=on  hw_selection=Fabric  pipelined=off  use_rpm=on  dbl_ovrd=off  block_type=addsub
      settings: xl_area=[0, 0, 0, 0, 0, 0, 0]  block_version=VER_STRING_GOES_HERE
  AddSub3 : xbsIndex_r4/AddSub  mode=Addition or Subtraction  use_carryin=off  use_carryout=off  en=off  latency=0  precision=User Defined  arith_type="Signed  (2's comp)"  n_bits=15  bin_pt=12  quantization=Truncate  overflow=Wrap  use_behavioral_HDL=on  hw_selection=Fabric  pipelined=off  use_rpm=on  dbl_ovrd=off  block_type=addsub
      settings: xl_area=[0, 0, 0, 0, 0, 0, 0]  block_version=VER_STRING_GOES_HERE
  Constant : xbsIndex_r4/Constant  const=atan(2^-i)  gui_display_data_type=Fixed-point  arith_type=Signed (2's comp)  n_bits=20  bin_pt=18  preci_type=Single  exp_width=8  frac_width=24  explicit_period=off  period=1  equ=P=C  opselect=C  inp2=PCIN>>17  opr=+  inp1=P  carry=CIN  dbl_ovrd=off  block_type=constant
      settings: block_version=10.1.2
  Inverter : xbsIndex_r4/Inverter  en=off  latency=0  dbl_ovrd=off  block_type=inv
      settings: xl_area=[0, 0, 0, 0, 0, 0, 0]  block_version=VER_STRING_GOES_HERE
  Logical : xbsIndex_r4/Logical  logical_function=XOR  inputs=2  en=off  latency=0  precision=Full  arith_type=Unsigned  n_bits=1  bin_pt=0  align_bp=on  dbl_ovrd=off  block_type=logical
      settings: xl_area=[0, 0, 0, 0, 0, 0, 0]  block_version=VER_STRING_GOES_HERE
  Shift : xbsIndex_r4/Shift  shift_dir=Right  shift_bits=i  en=off  latency=0  precision=User Defined  arith_type="Signed  (2's comp)"  n_bits=15  bin_pt=12  quantization=Truncate  overflow=Wrap  dbl_ovrd=off  block_type=shift
      settings: xl_area=[0, 0, 0, 0, 0, 0, 0]  block_version=VER_STRING_GOES_HERE
  Shift1 : xbsIndex_r4/Shift  shift_dir=Right  shift_bits=i  en=off  latency=0  precision=User Defined  arith_type="Signed  (2's comp)"  n_bits=15  bin_pt=12  quantization=Truncate  overflow=Wrap  dbl_ovrd=off  block_type=shift
      settings: xl_area=[0, 0, 0, 0, 0, 0, 0]  block_version=VER_STRING_GOES_HERE
  Slice : xbsIndex_r4/Slice  nbits=1  boolean_output=on  mode=Upper Bit Location + Width  bit1=0  base1=MSB of Input  bit0=0  base0=LSB of Input  dbl_ovrd=off  block_type=slice
      settings: infoedit="Extracts a given range of bits from each input sample and presents it at the output.  The output type is ordinarily unsigned with binary point at zero, but can be Boolean when the slice is one bit wide.<P><P>Hardware notes: In hardware this block costs nothing."  block_version=VER_STRING_GOES_HERE
  Slice1 : xbsIndex_r4/Slice  nbits=1  boolean_output=on  mode=Upper Bit Location + Width  bit1=0  base1=MSB of Input  bit0=0  base0=LSB of Input  dbl_ovrd=off  block_type=slice
      settings: infoedit="Extracts a given range of bits from each input sample and presents it at the output.  The output type is ordinarily unsigned with binary point at zero, but can be Boolean when the slice is one bit wide.<P><P>Hardware notes: In hardware this block costs nothing."  block_version=VER_STRING_GOES_HERE
  x out : Outport
  y out : Outport  Port=2
  z out : Outport  Port=3
  wires:
  x in/1 -> AddSub2/1, Shift/1, Slice/1
  y in/1 -> AddSub3/1, Shift1/1, Slice1/1
  Slice/1 -> Logical/1
  Slice1/1 -> Logical/2
  Logical/1 -> Inverter/1, AddSub2/3, AddSub1/3
  Shift1/1 -> AddSub2/2
  Shift/1 -> AddSub3/2
  Inverter/1 -> AddSub3/3
  AddSub2/1 -> x out/1
  AddSub3/1 -> y out/1
  z in/1 -> AddSub1/1
  Constant/1 -> AddSub1/2
  AddSub1/1 -> z out/1
